simulink library "ServoModel"  (R2014b)
settings: Solver=ode45  StartTime=0.0  StopTime=10.0  RelTol=1e-3
undefined symbols (not defined in the file): D, I, N, P, satvel
libraries: ServoModel x12, simulink x2, simulink_extras x1
settings Model: Creator=Sebastian  LastModifiedBy=Sebastian

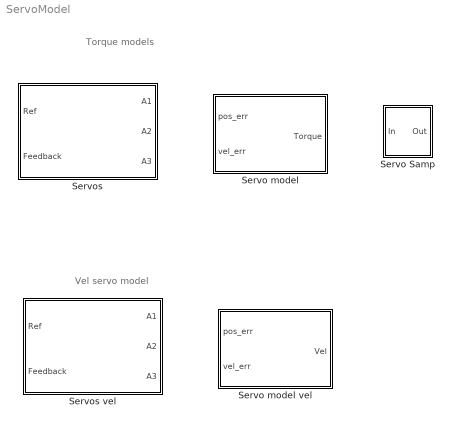
== system ServoModel ==
  note: Vel servo model
  note: Torque models
  Servo Samp : Subsystem
  Servo model : Subsystem
  Servo model vel : Subsystem
  Servos : Subsystem
  Servos vel : Subsystem

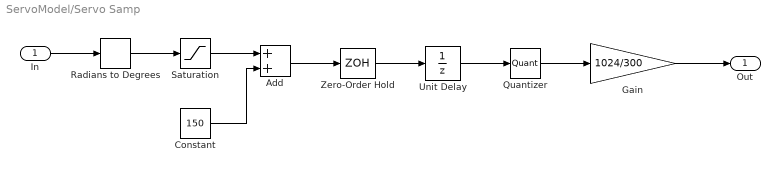
== system ServoModel/Servo Samp ==
  In : Inport
  Add : Sum
  Constant : Constant  Value=150  SampleTime=0.001
  Gain : Gain  Gain=1024/300
  Quantizer : Quantizer  QuantizationInterval=300/1024
  Radians to Degrees : simulink_extras/Transformations/Radians to Degrees
  Saturation : Saturate  UpperLimit=150  LowerLimit=-150
  Unit Delay : UnitDelay  InitialCondition=150  SampleTime=-1
  Zero-Order Hold : ZeroOrderHold  SampleTime=0.001
  Out : Outport
  wires:
  Quantizer/1 -> Gain/1
  Radians to Degrees/1 -> Saturation/1
  Add/1 -> Zero-Order Hold/1
  Gain/1 -> Out/1
  Constant/1 -> Add/2
  In/1 -> Radians to Degrees/1
  Unit Delay/1 -> Quantizer/1
  Saturation/1 -> Add/1
  Zero-Order Hold/1 -> Unit Delay/1

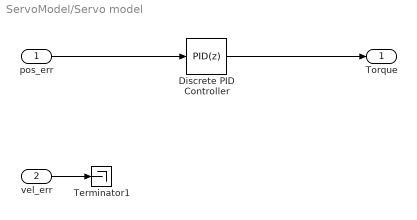
== system ServoModel/Servo model ==
  pos_err : Inport
  vel_err : Inport  Port=2
  Discrete PID Controller : simulink/Continuous/PID Controller  Controller=PID  TimeDomain=Discrete-time  SampleTime=0.001  IntegratorMethod=Backward Euler  FilterMethod=Forward Euler  Form=Parallel  P=0.00413190191601698  I=0.00483915491408406  D=-0.000158697423692473  N=11.6663153258342  InitialConditionSource=internal  InitialConditionForIntegrator=0  InitialConditionForFilter=0  ExternalReset=none  IgnoreLimit=on  LimitOutput=off  UpperSaturationLimit=1.5  LowerSaturationLimit=-1.5  LinearizeAsGain=off  AntiWindupMode=clamping  Kb=1  TrackingMode=off  Kt=1  PParamMin=[]  PParamMax=[]  IParamMin=[]  IParamMax=[]  DParamMin=[]  DParamMax=[]  NParamMin=[]  NParamMax=[]  KbParamMin=[]  KbParamMax=[]  KtParamMin=[]  KtParamMax=[]  POutMin=[]  POutMax=[]  IOutMin=[]  IOutMax=[]  DOutMin=[]  DOutMax=[]  NOutMin=[]  NOutMax=[]  KbOutMin=[]  KbOutMax=[]  KtOutMin=[]  KtOutMax=[]  IntegratorOutMin=[]  IntegratorOutMax=[]  FilterOutMin=[]  FilterOutMax=[]  SumOutMin=[]  SumOutMax=[]  SumI1OutMin=[]  SumI1OutMax=[]  SumI2OutMin=[]  SumI2OutMax=[]  SumI3OutMin=[]  SumI3OutMax=[]  SumDOutMin=[]  SumDOutMax=[]  SaturationOutMin=[]  SaturationOutMax=[]  IntegratorContinuousStateAttributes=''  IntegratorStateMustResolveToSignalObject=off  IntegratorRTWStateStorageClass=Auto  FilterContinuousStateAttributes=''  FilterStateMustResolveToSignalObject=off  FilterRTWStateStorageClass=Auto  DifferentiatorICPrevScaledInput=0  DifferentiatorOutMin=[]  DifferentiatorOutMax=[]  UseFilter=on
  Terminator1 : Terminator
  Torque : Outport
  wires:
  vel_err/1 -> Terminator1/1
  pos_err/1 -> Discrete PID Controller/1
  Discrete PID Controller/1 -> Torque/1

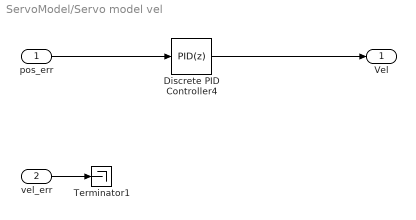
== system ServoModel/Servo model vel ==
  pos_err : Inport
  vel_err : Inport  Port=2
  Discrete PID Controller4 : simulink/Continuous/PID Controller  Controller=PID  TimeDomain=Discrete-time  SampleTime=0.01  IntegratorMethod=Forward Euler  FilterMethod=Forward Euler  Form=Parallel  P=P  I=I  D=D  N=N  InitialConditionSource=internal  InitialConditionForIntegrator=0  InitialConditionForFilter=0  ExternalReset=none  IgnoreLimit=on  LimitOutput=on  UpperSaturationLimit=satvel  LowerSaturationLimit=-satvel  LinearizeAsGain=off  AntiWindupMode=clamping  Kb=1  TrackingMode=off  Kt=1  PParamMin=[]  PParamMax=[]  IParamMin=[]  IParamMax=[]  DParamMin=[]  DParamMax=[]  NParamMin=[]  NParamMax=[]  KbParamMin=[]  KbParamMax=[]  KtParamMin=[]  KtParamMax=[]  POutMin=[]  POutMax=[]  IOutMin=[]  IOutMax=[]  DOutMin=[]  DOutMax=[]  NOutMin=[]  NOutMax=[]  KbOutMin=[]  KbOutMax=[]  KtOutMin=[]  KtOutMax=[]  IntegratorOutMin=[]  IntegratorOutMax=[]  FilterOutMin=[]  FilterOutMax=[]  SumOutMin=[]  SumOutMax=[]  SumI1OutMin=[]  SumI1OutMax=[]  SumI2OutMin=[]  SumI2OutMax=[]  SumI3OutMin=[]  SumI3OutMax=[]  SumDOutMin=[]  SumDOutMax=[]  SaturationOutMin=[]  SaturationOutMax=[]  IntegratorContinuousStateAttributes=''  IntegratorStateMustResolveToSignalObject=off  IntegratorRTWStateStorageClass=Auto  FilterContinuousStateAttributes=''  FilterStateMustResolveToSignalObject=off  FilterRTWStateStorageClass=Auto  DifferentiatorICPrevScaledInput=0  DifferentiatorOutMin=[]  DifferentiatorOutMax=[]  UseFilter=on
  Terminator1 : Terminator
  Vel : Outport
  wires:
  vel_err/1 -> Terminator1/1
  pos_err/1 -> Discrete PID Controller4/1
  Discrete PID Controller4/1 -> Vel/1

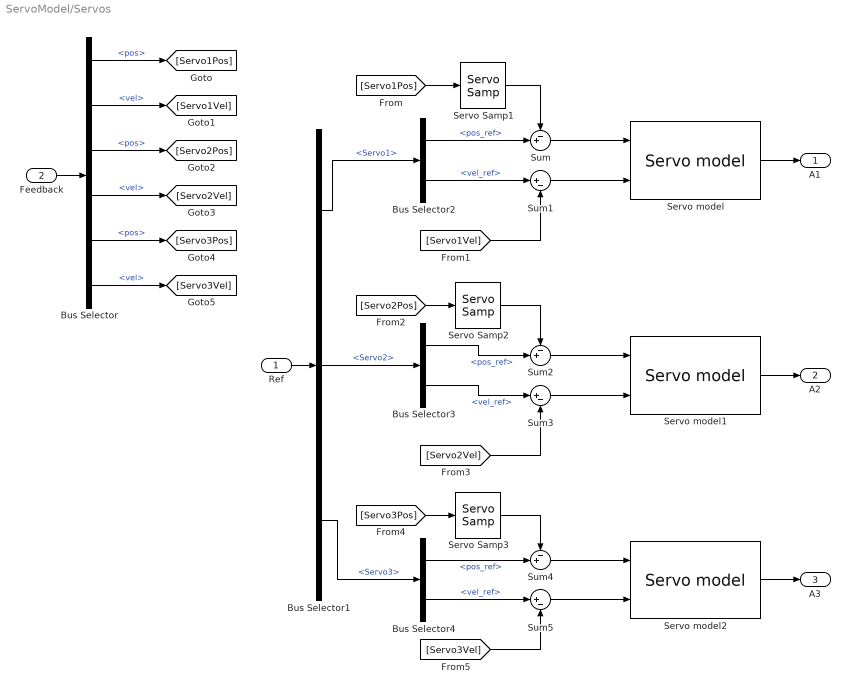
== system ServoModel/Servos ==
  Ref : Inport  OutDataTypeStr=Bus: Leg_ref
  Feedback : Inport  Port=2  OutDataTypeStr=Bus: Leg_mes  PortDimensions=3
  Bus Selector : BusSelector  OutputSignals=Servo1.pos,Servo1.vel,Servo2.pos,Servo2.vel,Servo3.pos,Servo3.vel
  Bus Selector1 : BusSelector  OutputSignals=Servo1,Servo2,Servo3
  Bus Selector2 : BusSelector  OutputSignals=pos_ref,vel_ref
  Bus Selector3 : BusSelector  OutputSignals=pos_ref,vel_ref
  Bus Selector4 : BusSelector  OutputSignals=pos_ref,vel_ref
  Servo Samp1 : ServoModel/Servo Samp
  Servo Samp2 : ServoModel/Servo Samp
  Servo Samp3 : ServoModel/Servo Samp
  Servo model : ServoModel/Servo model
  Servo model1 : ServoModel/Servo model
  Servo model2 : ServoModel/Servo model
  Sum : Sum  Inputs=-+|
  Sum1 : Sum  Inputs=|+-
  Sum2 : Sum  Inputs=-+|
  Sum3 : Sum  Inputs=|+-
  Sum4 : Sum  Inputs=-+|
  Sum5 : Sum  Inputs=|+-
  A1 : Outport
  A2 : Outport  Port=2
  A3 : Outport  Port=3
  wires:
  Ref/1 -> Bus Selector1/1
  Servo model/1 -> A1/1
  Bus Selector1/1 -> Bus Selector2/1  "<Servo1>"
  Bus Selector2/1 -> Sum/2  "<pos_ref>"
  Sum1/1 -> Servo model/2
  Sum/1 -> Servo model/1
  Servo model1/1 -> A2/1
  Sum3/1 -> Servo model1/2
  Sum2/1 -> Servo model1/1
  Servo model2/1 -> A3/1
  Sum5/1 -> Servo model2/2
  Sum4/1 -> Servo model2/1
  Bus Selector4/2 -> Sum5/1  "<vel_ref>"
  Bus Selector1/3 -> Bus Selector4/1  "<Servo3>"
  Bus Selector1/2 -> Bus Selector3/1  "<Servo2>"
  Feedback/1 -> Bus Selector/1
  Bus Selector/1 -> [Servo1Pos]  "<pos>"
  Bus Selector/2 -> [Servo1Vel]  "<vel>"
  Bus Selector/3 -> [Servo2Pos]  "<pos>"
  Bus Selector/4 -> [Servo2Vel]  "<vel>"
  Bus Selector/5 -> [Servo3Pos]  "<pos>"
  Bus Selector/6 -> [Servo3Vel]  "<vel>"
  [Servo1Vel] -> Sum1/2
  [Servo1Pos] -> Servo Samp1/1
  [Servo2Pos] -> Servo Samp2/1
  [Servo2Vel] -> Sum3/2
  [Servo3Pos] -> Servo Samp3/1
  [Servo3Vel] -> Sum5/2
  Bus Selector2/2 -> Sum1/1  "<vel_ref>"
  Bus Selector3/1 -> Sum2/2  "<pos_ref>"
  Bus Selector3/2 -> Sum3/1  "<vel_ref>"
  Bus Selector4/1 -> Sum4/2  "<pos_ref>"
  Servo Samp1/1 -> Sum/1
  Servo Samp2/1 -> Sum2/1
  Servo Samp3/1 -> Sum4/1

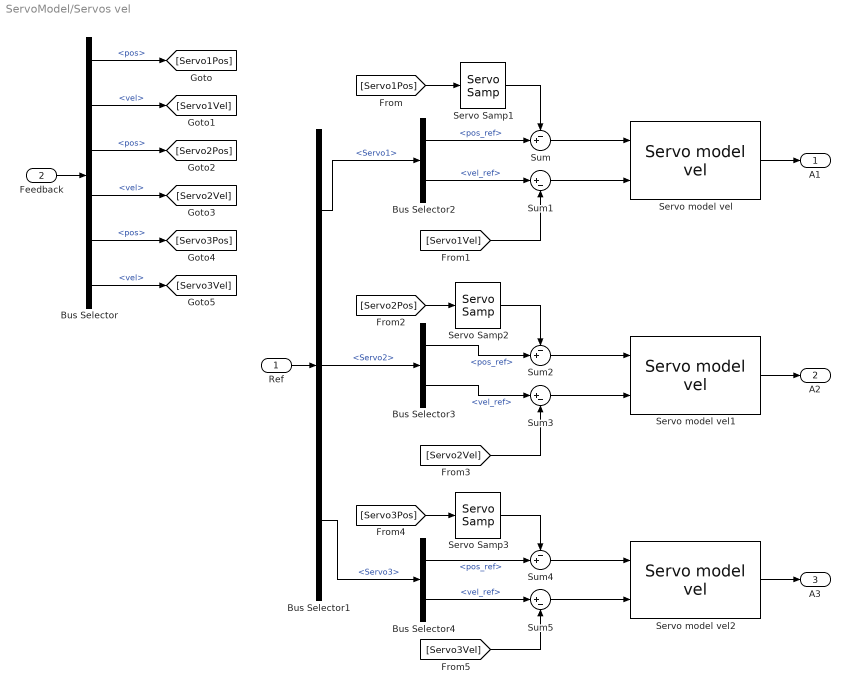
== system ServoModel/Servos vel ==
  Ref : Inport  OutDataTypeStr=Bus: Leg_ref
  Feedback : Inport  Port=2  OutDataTypeStr=Bus: Leg_mes  PortDimensions=3
  Bus Selector : BusSelector  OutputSignals=Servo1.pos,Servo1.vel,Servo2.pos,Servo2.vel,Servo3.pos,Servo3.vel
  Bus Selector1 : BusSelector  OutputSignals=Servo1,Servo2,Servo3
  Bus Selector2 : BusSelector  OutputSignals=pos_ref,vel_ref
  Bus Selector3 : BusSelector  OutputSignals=pos_ref,vel_ref
  Bus Selector4 : BusSelector  OutputSignals=pos_ref,vel_ref
  Servo Samp1 : ServoModel/Servo Samp
  Servo Samp2 : ServoModel/Servo Samp
  Servo Samp3 : ServoModel/Servo Samp
  Servo model vel : ServoModel/Servo model vel
  Servo model vel1 : ServoModel/Servo model vel
  Servo model vel2 : ServoModel/Servo model vel
  Sum : Sum  Inputs=-+|
  Sum1 : Sum  Inputs=|+-
  Sum2 : Sum  Inputs=-+|
  Sum3 : Sum  Inputs=|+-
  Sum4 : Sum  Inputs=-+|
  Sum5 : Sum  Inputs=|+-
  A1 : Outport
  A2 : Outport  Port=2
  A3 : Outport  Port=3
  wires:
  Ref/1 -> Bus Selector1/1
  Servo model vel/1 -> A1/1
  Bus Selector1/1 -> Bus Selector2/1  "<Servo1>"
  Bus Selector2/1 -> Sum/2  "<pos_ref>"
  Sum1/1 -> Servo model vel/2
  Sum/1 -> Servo model vel/1
  Servo model vel1/1 -> A2/1
  Sum3/1 -> Servo model vel1/2
  Sum2/1 -> Servo model vel1/1
  Servo model vel2/1 -> A3/1
  Sum5/1 -> Servo model vel2/2
  Sum4/1 -> Servo model vel2/1
  Bus Selector4/2 -> Sum5/1  "<vel_ref>"
  Bus Selector1/3 -> Bus Selector4/1  "<Servo3>"
  Bus Selector1/2 -> Bus Selector3/1  "<Servo2>"
  Feedback/1 -> Bus Selector/1
  Bus Selector/1 -> [Servo1Pos]  "<pos>"
  Bus Selector/2 -> [Servo1Vel]  "<vel>"
  Bus Selector/3 -> [Servo2Pos]  "<pos>"
  Bus Selector/4 -> [Servo2Vel]  "<vel>"
  Bus Selector/5 -> [Servo3Pos]  "<pos>"
  Bus Selector/6 -> [Servo3Vel]  "<vel>"
  [Servo1Vel] -> Sum1/2
  [Servo1Pos] -> Servo Samp1/1
  [Servo2Pos] -> Servo Samp2/1
  [Servo2Vel] -> Sum3/2
  [Servo3Pos] -> Servo Samp3/1
  [Servo3Vel] -> Sum5/2
  Bus Selector2/2 -> Sum1/1  "<vel_ref>"
  Bus Selector3/1 -> Sum2/2  "<pos_ref>"
  Bus Selector3/2 -> Sum3/1  "<vel_ref>"
  Bus Selector4/1 -> Sum4/2  "<pos_ref>"
  Servo Samp1/1 -> Sum/1
  Servo Samp2/1 -> Sum2/1
  Servo Samp3/1 -> Sum4/1
